simulink model "test_katadc_inter"  (Simulink 7.2)
settings: Solver=ode45  StartTime=0.0  StopTime=10.0  RelTol=1e-3
libraries: xbsIndex_r4 x244, simulink x29, dspsigops x12, casper_library_misc x3, xps_library x1
(part 2 of 2)

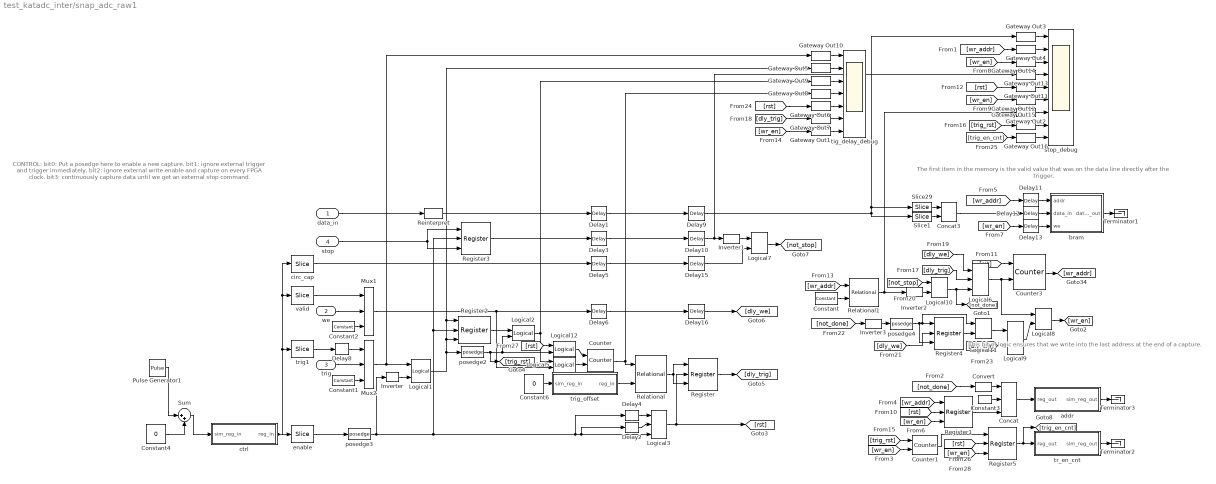
== system test_katadc_inter/snap_adc_raw1 ==
  note: This bit of logic ensures that we
      | write into the last address
      | at the end of a capture.
  note: The first item in the memory
      | is the valid value that was on the
      | data line directly after the trigger.
  note: CONTROL:
      | bit0: Put a posedge here to enable a new capture.
      | bit1: ignore external trigger and trigger immediately.
      | bit2: ignore external write enable and capture on every FPGA clock.
      | bit3: continuously capture data until we get an external stop command.
  data_in : Inport  OutDataType=sfix(16)  OutScaling=2^0
  we : Inport  Port=2  OutDataType=sfix(16)  OutScaling=2^0
  trig : Inport  Port=3  OutDataType=sfix(16)  OutScaling=2^0
  stop : Inport  Port=4  OutDataType=sfix(16)  OutScaling=2^0
  Concat : xbsIndex_r4/Concat  num_inputs=3  dbl_ovrd=off  block_type=concat
      settings: block_version=10.1.3
  Concat3 : xbsIndex_r4/Concat  num_inputs=2  dbl_ovrd=off  block_type=concat
      settings: block_version=10.1.3
  Constant : xbsIndex_r4/Constant  arith_type=Unsigned  const=(2^nsamples)-1  n_bits=nsamples  bin_pt=0  explicit_period=on  period=1  equ=P=C  opselect=C  inp2=PCIN>>17  opr=+  inp1=P  carry=CIN  dbl_ovrd=off  block_type=constant
  Constant1 : xbsIndex_r4/Constant  arith_type=Boolean  const=1  n_bits=1  bin_pt=0  explicit_period=on  period=1  equ=P=C  opselect=C  inp2=PCIN>>17  opr=+  inp1=P  carry=CIN  dbl_ovrd=off  block_type=constant
  Constant2 : xbsIndex_r4/Constant  arith_type=Boolean  const=1  n_bits=1  bin_pt=0  explicit_period=on  period=1  equ=P=C  opselect=C  inp2=PCIN>>17  opr=+  inp1=P  carry=CIN  dbl_ovrd=off  block_type=constant
  Constant3 : xbsIndex_r4/Constant  arith_type=Unsigned  const=0  n_bits=32-nsamples-1  bin_pt=0  explicit_period=on  period=1  equ=P=C  opselect=C  inp2=PCIN>>17  opr=+  inp1=P  carry=CIN  dbl_ovrd=off  block_type=constant
  Constant4 : Constant  Value=0  OutDataType=sfix(16)  OutScaling=2^0
  Constant6 : Constant  Value=0  OutDataType=sfix(16)  OutScaling=2^0
  Convert : xbsIndex_r4/Convert  arith_type=Unsigned  n_bits=1  bin_pt=0  quantization=Truncate  overflow=Wrap  latency=0  dbl_ovrd=off  pipeline=off  block_type=convert
      settings: block_version=10.1.3
  Counter : xbsIndex_r4/Counter  cnt_type=Free Running  cnt_to=Inf  operation=Up  start_count=0  cnt_by_val=1  arith_type=Unsigned  n_bits=32  bin_pt=0  load_pin=off  rst=on  en=on  explicit_period=on  period=1  dbl_ovrd=off  use_behavioral_HDL=off  implementation=Fabric  use_rpm=on  block_type=counter
      settings: xl_area=[0, 0, 0, 0, 0, 0, 0]
  Counter1 : xbsIndex_r4/Counter  cnt_type=Free Running  cnt_to=Inf  operation=Up  start_count=0  cnt_by_val=1  arith_type=Unsigned  n_bits=32  bin_pt=0  load_pin=off  rst=on  en=on  explicit_period=on  period=1  dbl_ovrd=off  use_behavioral_HDL=off  implementation=Fabric  use_rpm=on  block_type=counter
      settings: xl_area=[0, 0, 0, 0, 0, 0, 0]
  Counter3 : xbsIndex_r4/Counter  cnt_type=Free Running  cnt_to=1  operation=Up  start_count=0  cnt_by_val=1  arith_type=Unsigned  n_bits=nsamples  bin_pt=0  load_pin=off  rst=on  en=on  explicit_period=on  period=1  dbl_ovrd=off  use_behavioral_HDL=off  implementation=Fabric  use_rpm=on  block_type=counter
      settings: xl_area=[0, 0, 0, 0, 0, 0, 0]
  Delay{1,3..6,9..13,15..16} (12 alike) : xbsIndex_r4/Delay  en=off  latency=1  dbl_ovrd=off  reg_retiming=on  block_type=delay
      settings: xl_area=[0, 0, 0, 0, 0, 0, 0]
  Delay2 : xbsIndex_r4/Delay  en=off  latency=2  dbl_ovrd=off  reg_retiming=on  block_type=delay
      settings: xl_area=[0, 0, 0, 0, 0, 0, 0]
  Delay8 : xbsIndex_r4/Delay  en=off  latency=3  dbl_ovrd=off  reg_retiming=on  block_type=delay
      settings: xl_area=[0, 0, 0, 0, 0, 0, 0]
  Gateway Out{1..16} (16 alike) : xbsIndex_r4/Gateway Out  hdl_port=off  timing_constraint=None  locs_specified=off  LOCs={}  block_type=gatewayout
      settings: infoedit="Gateway out block.  Converts Xilinx fixed point inputs into ouputs of type Simulink integer, double, or fixed point.<P><P>Hardware notes:  In hardware these blocks become top level output ports or are discarded, depending on how they are configured."  xl_area=[0, 0, 0, 0, 0, 0, 0]  block_version=10.1.3
  Inverter{,1..3} (4 alike) : xbsIndex_r4/Inverter  en=off  latency=0  dbl_ovrd=off  block_type=inv
      settings: xl_area=[0, 0, 0, 0, 0, 0, 0]
  Logical{1,5,7,9} (4 alike) : xbsIndex_r4/Logical  logical_function=AND  inputs=2  en=off  latency=0  precision=Full  arith_type=Unsigned  n_bits=8  bin_pt=2  align_bp=on  dbl_ovrd=off  block_type=logical
      settings: xl_area=[0, 0, 0, 0, 0, 0, 0]
  Logical{2,8,10..12} (5 alike) : xbsIndex_r4/Logical  logical_function=OR  inputs=2  en=off  latency=0  precision=Full  arith_type=Unsigned  n_bits=8  bin_pt=2  align_bp=on  dbl_ovrd=off  block_type=logical
      settings: xl_area=[0, 0, 0, 0, 0, 0, 0]
  Logical3 : xbsIndex_r4/Logical  logical_function=OR  inputs=3  en=off  latency=0  precision=Full  arith_type=Unsigned  n_bits=8  bin_pt=2  align_bp=on  dbl_ovrd=off  block_type=logical
      settings: xl_area=[0, 0, 0, 0, 0, 0, 0]
  Logical6 : xbsIndex_r4/Logical  logical_function=AND  inputs=3  en=off  latency=0  precision=Full  arith_type=Unsigned  n_bits=8  bin_pt=2  align_bp=on  dbl_ovrd=off  block_type=logical
      settings: xl_area=[0, 0, 0, 0, 0, 0, 0]
  Mux1 : xbsIndex_r4/Mux  inputs=2  en=off  latency=0  precision=Full  arith_type="Signed  (2's comp)"  n_bits=8  bin_pt=2  quantization=Truncate  overflow=Wrap  dbl_ovrd=off  block_type=mux
      settings: xl_area=[0, 0, 0, 0, 0, 0, 0]
  Mux2 : xbsIndex_r4/Mux  inputs=2  en=off  latency=0  precision=Full  arith_type="Signed  (2's comp)"  n_bits=8  bin_pt=2  quantization=Truncate  overflow=Wrap  dbl_ovrd=off  block_type=mux
      settings: xl_area=[0, 0, 0, 0, 0, 0, 0]
  Pulse Generator1 : DiscretePulseGenerator  Period=2^(nsamples+2)  PulseWidth=2
  Register{,1..5} (6 alike) : xbsIndex_r4/Register  init=0  rst=on  en=on  dbl_ovrd=off  block_type=register
      settings: xl_area=[0, 0, 0, 0, 0, 0, 0]
  Reinterpret : xbsIndex_r4/Reinterpret  force_arith_type=on  arith_type=Unsigned  force_bin_pt=on  bin_pt=0  block_type=reinterpret
      settings: infoedit="Changes signal type without altering the binary representation.   You can changed the signal between signed and unsigned, and relocate the binary point.<P><P>Hardware notes: In hardware this block costs nothing.<P><P>Example:  Suppose the input is 6 bits wide, signed, with 2 fractional bits, and the output is forced to unsigned with 0 fractional bits.  Then an input of -2.0 (1110.00 in binary 2's complement) becomes an output of 56 (111000 in binary)."  block_version=10.1.3
  Relational : xbsIndex_r4/Relational  mode=a>b  en=off  latency=0  dbl_ovrd=off  block_type=relational
      settings: xl_area=[0, 0, 0, 0, 0, 0, 0]  block_version=10.1.3
  Relational1 : xbsIndex_r4/Relational  mode=a>=b  en=off  latency=0  dbl_ovrd=off  block_type=relational
      settings: xl_area=[0, 0, 0, 0, 0, 0, 0]  block_version=10.1.3
  Slice1 : xbsIndex_r4/Slice  nbits=32  boolean_output=off  mode=Upper Bit Location + Width  bit1=0  base1=MSB of Input  bit0=0  base0=LSB of Input  dbl_ovrd=off  block_type=slice
  Slice29 : xbsIndex_r4/Slice  nbits=32  boolean_output=off  mode=Lower Bit Location + Width  bit1=0  base1=MSB of Input  bit0=0  base0=LSB of Input  dbl_ovrd=off  block_type=slice
  Sum : Sum  Inputs=|++  OutDataType=sfix(16)  OutScaling=2^0
  Terminator1 : Terminator
  Terminator2 : Terminator
  Terminator3 : Terminator
  addr : Subsystem  Tag=xps:sw_reg  mask{io_dir=To Processor, arith_type=Unsigned, bitwidth=32, bin_pt=0, sample_period=1, latency=0}
      link override convert: arith_type=Unsigned  n_bits=32  bin_pt=0
      mask prompts: io_dir "I/O direction"; arith_type "Data Type"; bitwidth "Data bitwidth"; bin_pt "Data binary point"; sample_period "Sample period"
      mask init:
      | gw_name = clear_name(gcb);
      | config.source = str2func('software_register_init');
      | config.toplevel = gcb;
      | xBlock( config, {io_dir, arith_type, bitwidth, bin_pt, ... 
      |     sample_period, gw_name, latency});
      mask StyleString: popup(From Processor|To Processor),popup(Unsigned|Signed  (2's comp)),edit,edit,edit,edit
  bram : Subsystem  Tag=xps:bram  AncestorBlock=xps_library/Shared BRAM  mask{arith_type=Unsigned, addr_width=nsamples, data_width=64, data_bin_pt=0, init_vals=0, sample_rate=1}
      mask prompts: arith_type "Output Data Type"; addr_width "Address width"; data_width "Data Width"; data_bin_pt "Data Binary Point"; init_vals "Initial values (simulation only)"; sample_rate "Sample rate"
      mask init:
      | shared_bram_mask;
      mask StyleString: popup(Unsigned|Signed  (2's comp)),edit,edit,edit,edit,edit
  circ_cap : xbsIndex_r4/Slice  nbits=1  boolean_output=on  mode=Lower Bit Location + Width  bit1=0  base1=LSB of Input  bit0=3  base0=LSB of Input  dbl_ovrd=off  block_type=slice
      settings: infoedit="Extracts a given range of bits from each input sample and presents it at the output.  The output type is ordinarily unsigned with binary point at zero, but can be Boolean when the slice is one bit wide.<P><P>Hardware notes: In hardware this block costs nothing."  block_version=10.1.3
  ctrl : Subsystem  Tag=xps:sw_reg  mask{io_dir=From Processor, arith_type=Unsigned, bitwidth=32, bin_pt=0, sample_period=1, latency=0}
      link override r_4f_2x_16a_r322d_snap_descramble0_ctrl_user_data_out: arith_type=Unsigned  n_bits=32  bin_pt=0  period=1
      link override test_snap2_10_1_snap_circ_ctrl_user_data_out: arith_type=Unsigned  n_bits=32  bin_pt=0  period=1
      link override test_snap_circ_snap_circ_ctrl_user_data_out: arith_type=Unsigned  n_bits=32  bin_pt=0  period=1
      mask prompts: io_dir "I/O direction"; arith_type "Data Type"; bitwidth "Data bitwidth"; bin_pt "Data binary point"; sample_period "Sample period"
      mask init:
      | gw_name = clear_name(gcb);
      | config.source = str2func('software_register_init');
      | config.toplevel = gcb;
      | xBlock( config, {io_dir, arith_type, bitwidth, bin_pt, ... 
      |     sample_period, gw_name, latency});
      mask StyleString: popup(From Processor|To Processor),popup(Unsigned|Signed  (2's comp)),edit,edit,edit,edit
  enable : xbsIndex_r4/Slice  nbits=1  boolean_output=on  mode=Lower Bit Location + Width  bit1=0  base1=LSB of Input  bit0=0  base0=LSB of Input  dbl_ovrd=off  block_type=slice
      settings: infoedit="Extracts a given range of bits from each input sample and presents it at the output.  The output type is ordinarily unsigned with binary point at zero, but can be Boolean when the slice is one bit wide.<P><P>Hardware notes: In hardware this block costs nothing."  block_version=10.1.3
  posedge2 : casper_library_misc/posedge  Tag=Rising Edge Detector  SystemSampleTime=-1
  posedge3 : casper_library_misc/posedge  Tag=Rising Edge Detector  SystemSampleTime=-1
  posedge4 : casper_library_misc/posedge  Tag=Rising Edge Detector  SystemSampleTime=-1
  stop_debug : Scope  NumInputPorts=9
      settings: YMin=2.72014e+008~0~0~-5~-5~-5~-5~-5~-5  YMax=3.00648e+008~110~1~5~5~5~5~5~5  SaveName=ScopeData12
  tig_delay_debug : Scope  NumInputPorts=7
      settings: YMin=2.72014e+008~0~0~-5~-5~-5~-5  YMax=3.00648e+008~110~1~5~5~5~5  SaveName=ScopeData16
  tr_en_cnt : Subsystem  Tag=xps:sw_reg  mask{io_dir=To Processor, arith_type=Unsigned, bitwidth=32, bin_pt=0, sample_period=1, latency=0}
      link override convert: arith_type=Unsigned  n_bits=32  bin_pt=0
      mask prompts: io_dir "I/O direction"; arith_type "Data Type"; bitwidth "Data bitwidth"; bin_pt "Data binary point"; sample_period "Sample period"
      mask init:
      | gw_name = clear_name(gcb);
      | config.source = str2func('software_register_init');
      | config.toplevel = gcb;
      | xBlock( config, {io_dir, arith_type, bitwidth, bin_pt, ... 
      |     sample_period, gw_name, latency});
      mask StyleString: popup(From Processor|To Processor),popup(Unsigned|Signed  (2's comp)),edit,edit,edit,edit
  trig1 : xbsIndex_r4/Slice  nbits=1  boolean_output=on  mode=Lower Bit Location + Width  bit1=0  base1=LSB of Input  bit0=1  base0=LSB of Input  dbl_ovrd=off  block_type=slice
      settings: infoedit="Extracts a given range of bits from each input sample and presents it at the output.  The output type is ordinarily unsigned with binary point at zero, but can be Boolean when the slice is one bit wide.<P><P>Hardware notes: In hardware this block costs nothing."  block_version=10.1.3
  trig_offset : Subsystem  Tag=xps:sw_reg  mask{io_dir=From Processor, arith_type=Unsigned, bitwidth=32, bin_pt=0, sample_period=1, latency=0}
      link override test_snap_circ_snap_circ_trig_offset_user_data_out: arith_type=Unsigned  n_bits=32  bin_pt=0  period=1
      mask prompts: io_dir "I/O direction"; arith_type "Data Type"; bitwidth "Data bitwidth"; bin_pt "Data binary point"; sample_period "Sample period"
      mask init:
      | gw_name = clear_name(gcb);
      | config.source = str2func('software_register_init');
      | config.toplevel = gcb;
      | xBlock( config, {io_dir, arith_type, bitwidth, bin_pt, ... 
      |     sample_period, gw_name, latency});
      mask StyleString: popup(From Processor|To Processor),popup(Unsigned|Signed  (2's comp)),edit,edit,edit,edit
  valid : xbsIndex_r4/Slice  nbits=1  boolean_output=on  mode=Lower Bit Location + Width  bit1=0  base1=LSB of Input  bit0=2  base0=LSB of Input  dbl_ovrd=off  block_type=slice
      settings: infoedit="Extracts a given range of bits from each input sample and presents it at the output.  The output type is ordinarily unsigned with binary point at zero, but can be Boolean when the slice is one bit wide.<P><P>Hardware notes: In hardware this block costs nothing."  block_version=10.1.3
  wires:
  Concat3/1 -> Delay12/1
  Slice1/1 -> Concat3/2
  Slice29/1 -> Concat3/1
  Delay6/1 -> Delay16/1
  Delay5/1 -> Delay15/1
  Delay3/1 -> Delay10/1
  Delay1/1 -> Delay9/1
  posedge2/1 -> [trig_rst], Logical12/2, Logical2/2
  [rst] -> Logical12/1
  Logical12/1 -> Counter/1
  Register5/1 -> tr_en_cnt/1(reg_out), [trig_en_cnt]
  [rst] -> Register5/2
  [wr_en] -> Register5/3
  Counter1/1 -> Register5/1
  Gateway Out16/1 -> stop_debug/9
  [trig_en_cnt] -> Gateway Out16/1
  Delay8/1 -> Mux2/1
  [rst] -> Gateway Out6/1
  Register4/1 -> Logical11/2
  Logical11/1 -> Logical9/1
  Logical9/1 -> Logical8/2
  [dly_we] -> Logical9/2
  [dly_we] -> Register4/2
  posedge4/1 -> Logical11/1, Register4/1, Register4/3
  Inverter3/1 -> posedge4/1
  [not_done] -> Inverter3/1
  Logical8/1 -> [wr_en]
  [not_stop] -> Logical10/1
  Logical7/1 -> [not_stop]
  [dly_trig] -> Logical6/2
  [dly_we] -> Logical6/1
  Delay16/1 -> [dly_we]
  [dly_trig] -> Gateway Out7/1
  Register/1 -> [dly_trig]
  [trig_rst] -> Gateway Out15/1
  Gateway Out15/1 -> stop_debug/8
  [trig_rst] -> Counter1/1
  [wr_en] -> Gateway Out1/1
  [wr_addr] -> Relational1/1
  Relational1/1 -> Inverter2/1, Gateway Out2/1
  [rst] -> Gateway Out11/1
  [rst] -> Counter3/1
  [rst] -> Register1/2
  [wr_en] -> Gateway Out12/1
  [wr_en] -> Gateway Out14/1
  [wr_en] -> Delay13/1
  [wr_en] -> Register1/3
  [wr_addr] -> Register1/1
  [wr_en] -> Counter1/2
  [not_done] -> Convert/1
  [wr_addr] -> Gateway Out4/1
  [wr_addr] -> Delay11/1
  Register1/1 -> Concat/3
  Logical5/1 -> Counter/2
  Delay15/1 -> Logical7/2
  Delay10/1 -> Gateway Out13/1, Inverter1/1
  Delay9/1 -> Slice1/1, Slice29/1, Gateway Out3/1
  bram/1(data_out) -> Terminator1/1
  addr/1(sim_reg_out) -> Terminator3/1
  tr_en_cnt/1(sim_reg_out) -> Terminator2/1
  Constant3/1 -> Concat/2
  Convert/1 -> Concat/1
  circ_cap/1 -> Delay5/1
  stop/1 -> Register3/3, Register3/1
  Concat/1 -> addr/1(reg_out)
  Delay13/1 -> bram/3(we)
  Delay12/1 -> bram/2(data_in)
  Delay11/1 -> bram/1(addr)
  Inverter2/1 -> Logical10/2
  Logical10/1 -> [not_done], Logical6/3
  Logical3/1 -> [rst], Register/2
  Gateway Out2/1 -> stop_debug/7
  Gateway Out12/1 -> stop_debug/6
  Gateway Out3/1 -> stop_debug/1
  Gateway Out11/1 -> stop_debug/5
  Gateway Out13/1 -> stop_debug/4
  Gateway Out4/1 -> stop_debug/2
  Gateway Out14/1 -> stop_debug/3
  Inverter1/1 -> Logical7/1
  Register3/1 -> Delay3/1
  Constant/1 -> Relational1/2
  Counter3/1 -> [wr_addr]
  Logical6/1 -> Logical8/1, Counter3/2
  Reinterpret/1 -> Delay1/1
  Gateway Out1/1 -> tig_delay_debug/7
  Gateway Out7/1 -> tig_delay_debug/6
  Gateway Out10/1 -> tig_delay_debug/1
  Gateway Out6/1 -> tig_delay_debug/5
  Gateway Out8/1 -> tig_delay_debug/4
  Gateway Out5/1 -> tig_delay_debug/2
  Gateway Out9/1 -> tig_delay_debug/3
  Delay2/1 -> Logical3/2
  Counter/1 -> Relational/1, Gateway Out8/1
  Logical2/1 -> Gateway Out9/1, Logical5/1
  Relational/1 -> Register/1, Register/3
  trig_offset/1(reg_in) -> Relational/2
  Constant6/1 -> trig_offset/1(sim_reg_in)
  Delay4/1 -> Logical3/1
  Register2/1 -> Logical2/1
  Logical1/1 -> posedge2/1, Register2/3, Gateway Out5/1, Register2/1
  posedge3/1 -> Register3/2, Register2/2, Logical3/3, Delay2/1, Delay4/1, Inverter/1
  Mux1/1 -> Delay6/1, Logical5/2
  Inverter/1 -> Logical1/2
  Mux2/1 -> Gateway Out10/1, Logical1/1
  Pulse Generator1/1 -> Sum/1
  Sum/1 -> ctrl/1(sim_reg_in)
  Constant4/1 -> Sum/2
  trig/1 -> Mux2/2
  enable/1 -> posedge3/1
  ctrl/1(reg_in) -> enable/1, circ_cap/1, valid/1, trig1/1
  Constant1/1 -> Mux2/3
  we/1 -> Mux1/2
  Constant2/1 -> Mux1/3
  trig1/1 -> Delay8/1
  valid/1 -> Mux1/1
  data_in/1 -> Reinterpret/1

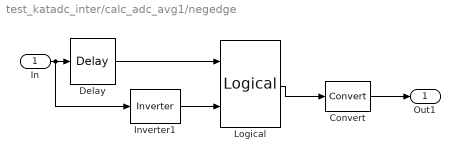
== system test_katadc_inter/calc_adc_avg1/negedge ==
  In : Inport  OutDataType=sfix(16)  OutScaling=2^0
  Convert : xbsIndex_r4/Convert  arith_type=Boolean  n_bits=8  bin_pt=6  quantization=Truncate  overflow=Wrap  latency=0  dbl_ovrd=off  pipeline=off  block_type=convert
      settings: xl_area=[0, 0, 0, 0, 0, 0, 0]  block_version=10.1.3
  Delay : xbsIndex_r4/Delay  en=off  latency=1  dbl_ovrd=off  reg_retiming=off  block_type=delay
      settings: xl_area=[0, 0, 0, 0, 0, 0, 0]
  Inverter1 : xbsIndex_r4/Inverter  en=off  latency=0  dbl_ovrd=off  block_type=inv
      settings: xl_area=[0, 0, 0, 0, 0, 0, 0]
  Logical : xbsIndex_r4/Logical  logical_function=AND  inputs=2  en=off  latency=0  precision=Full  arith_type=Unsigned  n_bits=8  bin_pt=2  align_bp=on  dbl_ovrd=off  block_type=logical
      settings: xl_area=[0, 0, 0, 0, 0, 0, 0]
  Out1 : Outport  OutDataType=sfix(16)  OutScaling=2^0
  wires:
  Inverter1/1 -> Logical/2
  Logical/1 -> Convert/1
  In/1 -> Inverter1/1, Delay/1
  Delay/1 -> Logical/1
  Convert/1 -> Out1/1

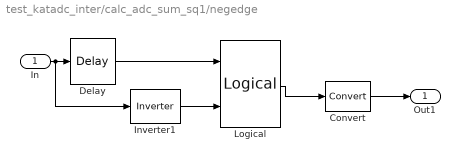
== system test_katadc_inter/calc_adc_sum_sq1/negedge ==
  In : Inport  OutDataType=sfix(16)  OutScaling=2^0
  Convert : xbsIndex_r4/Convert  arith_type=Boolean  n_bits=8  bin_pt=6  quantization=Truncate  overflow=Wrap  latency=0  dbl_ovrd=off  pipeline=off  block_type=convert
      settings: xl_area=[0, 0, 0, 0, 0, 0, 0]  block_version=10.1.3
  Delay : xbsIndex_r4/Delay  en=off  latency=1  dbl_ovrd=off  reg_retiming=off  block_type=delay
      settings: xl_area=[0, 0, 0, 0, 0, 0, 0]
  Inverter1 : xbsIndex_r4/Inverter  en=off  latency=0  dbl_ovrd=off  block_type=inv
      settings: xl_area=[0, 0, 0, 0, 0, 0, 0]
  Logical : xbsIndex_r4/Logical  logical_function=AND  inputs=2  en=off  latency=0  precision=Full  arith_type=Unsigned  n_bits=8  bin_pt=2  align_bp=on  dbl_ovrd=off  block_type=logical
      settings: xl_area=[0, 0, 0, 0, 0, 0, 0]
  Out1 : Outport  OutDataType=sfix(16)  OutScaling=2^0
  wires:
  Convert/1 -> Out1/1
  Delay/1 -> Logical/1
  In/1 -> Delay/1, Inverter1/1
  Logical/1 -> Convert/1
  Inverter1/1 -> Logical/2

== system test_katadc_inter/snap_adc_raw1/addr ==
  reg_out : Inport
  convert : xbsIndex_r4/Convert  arith_type=Unsigned  n_bits=32  bin_pt=0  quantization=Truncate  overflow=Wrap  latency=0  dbl_ovrd=off  pipeline=off  block_type=convert
      settings: block_version=11.4
  r_katadc_interleave_tests_snap_adc_raw1_addr_user_data_in : xbsIndex_r4/Gateway Out  hdl_port=on  timing_constraint=None  locs_specified=off  LOCs={}  block_type=gatewayout
      settings: infoedit="Gateway out block.  Converts Xilinx fixed point inputs into ouputs of type Simulink integer, double, or fixed point.<br><br>Hardware notes:  In hardware these blocks become top level output ports or are discarded, depending on how they are configured."  block_version=11.4
  sim_reg_out : Outport
  wires:
  r_katadc_interleave_tests_snap_adc_raw1_addr_user_data_in/1 -> sim_reg_out/1
  convert/1 -> r_katadc_interleave_tests_snap_adc_raw1_addr_user_data_in/1
  reg_out/1 -> convert/1

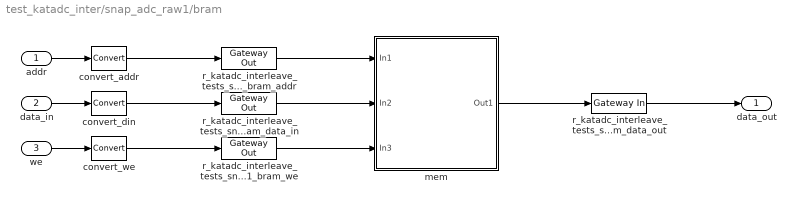
== system test_katadc_inter/snap_adc_raw1/bram ==
  addr : Inport  OutDataType=sfix(16)  OutScaling=2^0
  data_in : Inport  Port=2  OutDataType=sfix(16)  OutScaling=2^0
  we : Inport  Port=3  OutDataType=sfix(16)  OutScaling=2^0
  convert_addr : xbsIndex_r4/Convert  arith_type=Unsigned  n_bits=addr_width  bin_pt=0  quantization=Truncate  overflow=Wrap  latency=0  dbl_ovrd=off  pipeline=off  block_type=convert
      settings: xl_area=[0, 0, 0, 0, 0, 0, 0]
  convert_din : xbsIndex_r4/Convert  arith_type=Unsigned  n_bits=data_width  bin_pt=data_bin_pt  quantization=Truncate  overflow=Wrap  latency=0  dbl_ovrd=off  pipeline=off  block_type=convert
      settings: xl_area=[0, 0, 0, 0, 0, 0, 0]
  convert_we : xbsIndex_r4/Convert  arith_type=Unsigned  n_bits=1  bin_pt=0  quantization=Truncate  overflow=Wrap  latency=0  dbl_ovrd=off  pipeline=off  block_type=convert
      settings: xl_area=[0, 0, 0, 0, 0, 0, 0]
  mem : Subsystem
  r_katadc_interleave_tests_snap_adc_raw1_bram_addr : xbsIndex_r4/Gateway Out  hdl_port=on  timing_constraint=None  locs_specified=off  LOCs={'A5','B9','A9','C1','A3','G6','E9','A6','A7','A8','B8','B1','B3','D9','B5','B4','B6','C2'}  block_type=gatewayout
      settings: infoedit="Gateway out block.  Converts Xilinx fixed point inputs into ouputs of type Simulink integer, double, or fixed point.<P><P>Hardware notes:  In hardware these blocks become top level output ports or are discarded, depending on how they are configured."  xl_area=[0, 0, 0, 0, 0, 0, 0]  sginterface={'Nallatech'=>{'xdspkit'=>{'non_memory_mapped_port'=>'uprev_Shared_BRAM_addr'}},'Xilinx'=>{'jtaghwcosim'=>{'non_memory_mapped_port'=>'uprev_Shared_BRAM_addr'},'xdspkit'=>{'non_memory_mapped_port'=>'uprev_Shared_BRAM_addr'}}}
  r_katadc_interleave_tests_snap_adc_raw1_bram_data_in : xbsIndex_r4/Gateway Out  hdl_port=on  timing_constraint=None  locs_specified=off  LOCs={'B21','B22','A22','B23','B19','C19','A20','A21','A23','B24','A24','A25','E18','D18','C18','B18'}  block_type=gatewayout
      settings: infoedit="Gateway out block.  Converts Xilinx fixed point inputs into ouputs of type Simulink integer, double, or fixed point.<P><P>Hardware notes:  In hardware these blocks become top level output ports or are discarded, depending on how they are configured."  xl_area=[0, 0, 0, 0, 0, 0, 0]  sginterface={'Nallatech'=>{'xdspkit'=>{'non_memory_mapped_port'=>'uprev_Shared_BRAM_data_in'}},'Xilinx'=>{'jtaghwcosim'=>{'non_memory_mapped_port'=>'uprev_Shared_BRAM_data_in'},'xdspkit'=>{'non_memory_mapped_port'=>'uprev_Shared_BRAM_data_in'}}}
  r_katadc_interleave_tests_snap_adc_raw1_bram_data_out : xbsIndex_r4/Gateway In  arith_type=Unsigned  n_bits=data_width  bin_pt=data_bin_pt  quantization=Truncate  overflow=Wrap  period=sample_rate  dbl_ovrd=off  timing_constraint=None  locs_specified=off  LOCs={}  hdl_port=on  block_type=gatewayin
      settings: infoedit="Gateway in block.  Converts inputs of type Simulink integer, double and fixed point to  Xilinx fixed point type.<P><P>Hardware notes:  In hardware these blocks become top level input ports."  xl_area=[0, 0, 0, 0, 0, 0, 0]
  r_katadc_interleave_tests_snap_adc_raw1_bram_we : xbsIndex_r4/Gateway Out  hdl_port=on  timing_constraint=None  locs_specified=off  LOCs={'A14'}  block_type=gatewayout
      settings: infoedit="Gateway out block.  Converts Xilinx fixed point inputs into ouputs of type Simulink integer, double, or fixed point.<P><P>Hardware notes:  In hardware these blocks become top level output ports or are discarded, depending on how they are configured."  xl_area=[0, 0, 0, 0, 0, 0, 0]
  data_out : Outport  OutDataType=sfix(16)  OutScaling=2^0
  wires:
  mem/1(Out1) -> r_katadc_interleave_tests_snap_adc_raw1_bram_data_out/1
  data_in/1 -> convert_din/1
  r_katadc_interleave_tests_snap_adc_raw1_bram_data_out/1 -> data_out/1
  addr/1 -> convert_addr/1
  we/1 -> convert_we/1
  convert_addr/1 -> r_katadc_interleave_tests_snap_adc_raw1_bram_addr/1
  convert_we/1 -> r_katadc_interleave_tests_snap_adc_raw1_bram_we/1
  convert_din/1 -> r_katadc_interleave_tests_snap_adc_raw1_bram_data_in/1
  r_katadc_interleave_tests_snap_adc_raw1_bram_addr/1 -> mem/1(In1)
  r_katadc_interleave_tests_snap_adc_raw1_bram_data_in/1 -> mem/2(In2)
  r_katadc_interleave_tests_snap_adc_raw1_bram_we/1 -> mem/3(In3)

== system test_katadc_inter/snap_adc_raw1/ctrl ==
  sim_reg_in : Inport
  delay_pipe : Subsystem
  r_katadc_interleave_tests_snap_adc_raw1_ctrl_user_data_out : xbsIndex_r4/Gateway In  arith_type=Unsigned  n_bits=32  bin_pt=0  quantization="Round  (unbiased: +/- Inf)"  overflow=Saturate  period=1  dbl_ovrd=off  timing_constraint=None  locs_specified=off  LOCs={}  hdl_port=on  block_type=gatewayin
      settings: infoedit="Gateway in block.  Converts inputs of type Simulink integer, double and fixed point to  Xilinx fixed point type.<br><br>Hardware notes:  In hardware these blocks become top level input ports."  block_version=11.4
  reg_in : Outport
  wires:
  delay_pipe/1(q) -> reg_in/1
  r_katadc_interleave_tests_snap_adc_raw1_ctrl_user_data_out/1 -> delay_pipe/1(d)
  sim_reg_in/1 -> r_katadc_interleave_tests_snap_adc_raw1_ctrl_user_data_out/1

== system test_katadc_inter/snap_adc_raw1/tr_en_cnt ==
  reg_out : Inport
  convert : xbsIndex_r4/Convert  arith_type=Unsigned  n_bits=32  bin_pt=0  quantization=Truncate  overflow=Wrap  latency=0  dbl_ovrd=off  pipeline=off  block_type=convert
      settings: block_version=11.4
  r_katadc_interleave_tests_snap_adc_raw1_tr_en_cnt_user_data_in : xbsIndex_r4/Gateway Out  hdl_port=on  timing_constraint=None  locs_specified=off  LOCs={}  block_type=gatewayout
      settings: infoedit="Gateway out block.  Converts Xilinx fixed point inputs into ouputs of type Simulink integer, double, or fixed point.<br><br>Hardware notes:  In hardware these blocks become top level output ports or are discarded, depending on how they are configured."  block_version=11.4
  sim_reg_out : Outport
  wires:
  r_katadc_interleave_tests_snap_adc_raw1_tr_en_cnt_user_data_in/1 -> sim_reg_out/1
  convert/1 -> r_katadc_interleave_tests_snap_adc_raw1_tr_en_cnt_user_data_in/1
  reg_out/1 -> convert/1

== system test_katadc_inter/snap_adc_raw1/trig_offset ==
  sim_reg_in : Inport
  delay_pipe : Subsystem
  r_katadc_interleave_tests_snap_adc_raw1_trig_offset_user_data_out : xbsIndex_r4/Gateway In  arith_type=Unsigned  n_bits=32  bin_pt=0  quantization="Round  (unbiased: +/- Inf)"  overflow=Saturate  period=1  dbl_ovrd=off  timing_constraint=None  locs_specified=off  LOCs={}  hdl_port=on  block_type=gatewayin
      settings: infoedit="Gateway in block.  Converts inputs of type Simulink integer, double and fixed point to  Xilinx fixed point type.<br><br>Hardware notes:  In hardware these blocks become top level input ports."  block_version=11.4
  reg_in : Outport
  wires:
  delay_pipe/1(q) -> reg_in/1
  r_katadc_interleave_tests_snap_adc_raw1_trig_offset_user_data_out/1 -> delay_pipe/1(d)
  sim_reg_in/1 -> r_katadc_interleave_tests_snap_adc_raw1_trig_offset_user_data_out/1

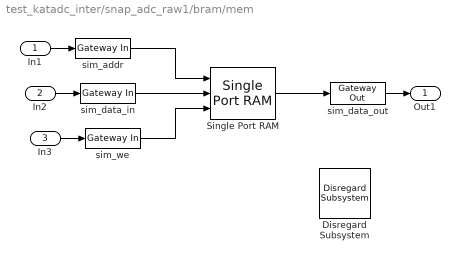
== system test_katadc_inter/snap_adc_raw1/bram/mem ==
  In1 : Inport  OutDataType=sfix(16)  OutScaling=2^0
  In2 : Inport  Port=2  OutDataType=sfix(16)  OutScaling=2^0
  In3 : Inport  Port=3  OutDataType=sfix(16)  OutScaling=2^0
  Disregard Subsystem : xbsIndex_r4/Disregard Subsystem  Tag=discardX  block_type=disregard
  Single Port RAM : xbsIndex_r4/Single Port RAM  depth=2^addr_width  initVector=init_vals  distributed_mem=Block RAM  write_mode=Read After Write  rst=off  init_reg=0  en=off  latency=1  dbl_ovrd=off  optimize=Area  use_rpm=off  block_type=spram
      settings: xl_area=[0, 0, 0, 0, 0, 0, 0]  block_version=9.1.01
  sim_addr : xbsIndex_r4/Gateway In  arith_type=Unsigned  n_bits=addr_width  bin_pt=0  quantization=Truncate  overflow=Wrap  period=sample_rate  dbl_ovrd=off  timing_constraint=None  locs_specified=off  LOCs={}  hdl_port=on  block_type=gatewayin
      settings: infoedit="Gateway in block.  Converts inputs of type Simulink integer, double and fixed point to  Xilinx fixed point type.<P><P>Hardware notes:  In hardware these blocks become top level input ports."  xl_area=[0, 0, 0, 0, 0, 0, 0]  sginterface={'Nallatech'=>{'xdspkit'=>{'non_memory_mapped_port'=>'sim_addr'}},'Xilinx'=>{'jtaghwcosim'=>{'non_memory_mapped_port'=>'sim_addr'},'xdspkit'=>{'non_memory_mapped_port'=>'sim_addr'}}}
  sim_data_in : xbsIndex_r4/Gateway In  arith_type=Unsigned  n_bits=data_width  bin_pt=data_bin_pt  quantization=Truncate  overflow=Wrap  period=sample_rate  dbl_ovrd=off  timing_constraint=None  locs_specified=off  LOCs={}  hdl_port=on  block_type=gatewayin
      settings: infoedit="Gateway in block.  Converts inputs of type Simulink integer, double and fixed point to  Xilinx fixed point type.<P><P>Hardware notes:  In hardware these blocks become top level input ports."  xl_area=[0, 0, 0, 0, 0, 0, 0]  sginterface={'Nallatech'=>{'xdspkit'=>{'non_memory_mapped_port'=>'sim_data_in'}},'Xilinx'=>{'jtaghwcosim'=>{'non_memory_mapped_port'=>'sim_data_in'},'xdspkit'=>{'non_memory_mapped_port'=>'sim_data_in'}}}
  sim_data_out : xbsIndex_r4/Gateway Out  hdl_port=on  timing_constraint=None  locs_specified=off  LOCs={'B21','B22','A22','B23','B19','C19','A20','A21','A23','B24','A24','A25','E18','D18','C18','B18'}  block_type=gatewayout
      settings: infoedit="Gateway out block.  Converts Xilinx fixed point inputs into ouputs of type Simulink integer, double, or fixed point.<P><P>Hardware notes:  In hardware these blocks become top level output ports or are discarded, depending on how they are configured."  xl_area=[0, 0, 0, 0, 0, 0, 0]  sginterface={'Nallatech'=>{'xdspkit'=>{'non_memory_mapped_port'=>'sim_data_out'}},'Xilinx'=>{'jtaghwcosim'=>{'non_memory_mapped_port'=>'sim_data_out'},'xdspkit'=>{'non_memory_mapped_port'=>'sim_data_out'}}}
  sim_we : xbsIndex_r4/Gateway In  arith_type=Boolean  n_bits=data_width  bin_pt=data_bin_pt  quantization=Truncate  overflow=Wrap  period=sample_rate  dbl_ovrd=off  timing_constraint=None  locs_specified=off  LOCs={}  hdl_port=on  block_type=gatewayin
      settings: infoedit="Gateway in block.  Converts inputs of type Simulink integer, double and fixed point to  Xilinx fixed point type.<P><P>Hardware notes:  In hardware these blocks become top level input ports."  xl_area=[0, 0, 0, 0, 0, 0, 0]  sginterface={'Nallatech'=>{'xdspkit'=>{'non_memory_mapped_port'=>'sim_we'}},'Xilinx'=>{'jtaghwcosim'=>{'non_memory_mapped_port'=>'sim_we'},'xdspkit'=>{'non_memory_mapped_port'=>'sim_we'}}}
  Out1 : Outport  OutDataType=sfix(16)  OutScaling=2^0
  wires:
  In3/1 -> sim_we/1
  sim_data_out/1 -> Out1/1
  In2/1 -> sim_data_in/1
  In1/1 -> sim_addr/1
  Single Port RAM/1 -> sim_data_out/1
  sim_we/1 -> Single Port RAM/3
  sim_data_in/1 -> Single Port RAM/2
  sim_addr/1 -> Single Port RAM/1

== system test_katadc_inter/snap_adc_raw1/ctrl/delay_pipe ==
  d : Inport
  q : Outport
  wires:
  d/1 -> q/1

== system test_katadc_inter/snap_adc_raw1/trig_offset/delay_pipe ==
  d : Inport
  q : Outport
  wires:
  d/1 -> q/1
